simulink model "linemodel"  (R2016a)
settings: Solver=VariableStepAuto  StartTime=0.0  StopTime=inf  RelTol=1e-3
undefined symbols (not defined in the file): A, B, C, D
libraries: simulink x4
settings Model: Creator=Gray  LastModifiedBy=Gray

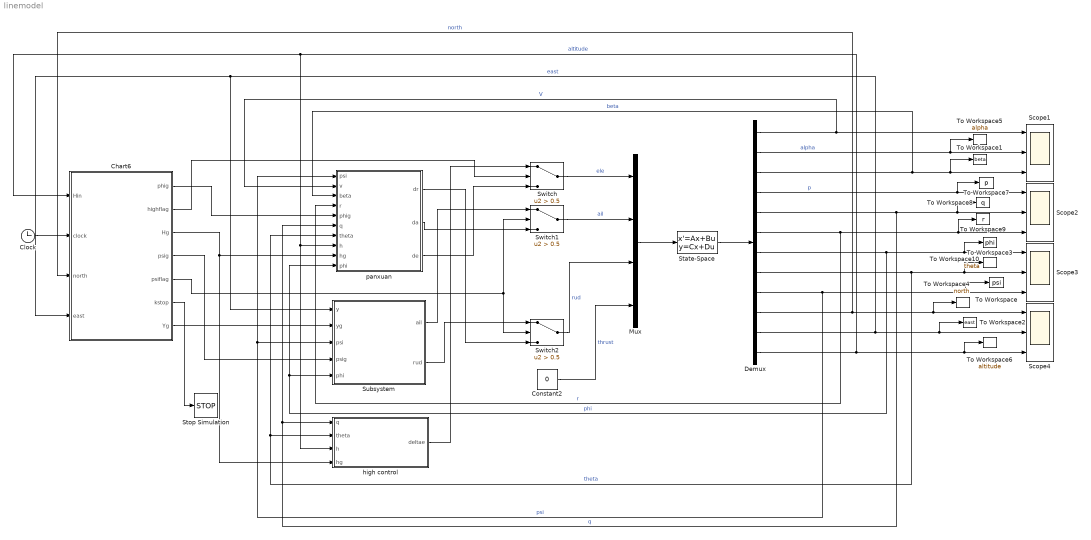
== system linemodel ==
  Chart6 : Stateflow chart  TreatAsAtomicUnit=on
  Clock : Clock
  Constant2 : Constant  Value=0
  Demux : Demux  Outputs=12
  Mux : Mux
  Scope{1..4} (4 alike) : Scope  NumInputPorts=3
  State-Space : StateSpace  A=A  B=B  C=C  D=D  X0=[20 0 0 0 0 0 0 0 0 0 0 0]
  Stop Simulation : Stop
  Subsystem : Subsystem
  Switch : Switch  Criteria=u2 > Threshold  Threshold=0.5
  Switch1 : Switch  Criteria=u2 > Threshold  Threshold=0.5
  Switch2 : Switch  Criteria=u2 > Threshold  Threshold=0.5
  To Workspace : ToWorkspace  VariableName=psi  SaveFormat=Timeseries  SampleTime=-1
  To Workspace1 : ToWorkspace  VariableName=beta  SaveFormat=Timeseries  SampleTime=-1
  To Workspace10 : ToWorkspace  VariableName=theta  SaveFormat=Timeseries  SampleTime=-1
  To Workspace2 : ToWorkspace  VariableName=east  SampleTime=-1
  To Workspace3 : ToWorkspace  VariableName=phi  SaveFormat=Timeseries  SampleTime=-1
  To Workspace4 : ToWorkspace  VariableName=north  SampleTime=-1
  To Workspace5 : ToWorkspace  VariableName=alpha  SaveFormat=Timeseries  SampleTime=-1
  To Workspace6 : ToWorkspace  VariableName=altitude  SaveFormat=Timeseries  SampleTime=-1
      settings: Save2DSignal=2-D array (concatenate along first dimension)
  To Workspace7 : ToWorkspace  VariableName=p  SaveFormat=Timeseries  SampleTime=-1
  To Workspace8 : ToWorkspace  VariableName=q  SaveFormat=Timeseries  SampleTime=-1
  To Workspace9 : ToWorkspace  VariableName=r  SaveFormat=Timeseries  SampleTime=-1
  high control : Subsystem
  panxuan : Subsystem
  wires:
  State-Space/1 -> Demux/1
  Mux/1 -> State-Space/1
  Demux/1 -> panxuan/2(v), Scope1/1  "V"
  Demux/2 -> To Workspace5/1, Scope1/2  "alpha"
  Demux/3 -> panxuan/3(beta), To Workspace1/1, Scope1/3  "beta"
  Demux/4 -> To Workspace7/1, Scope2/1  "p"
  Demux/5 -> panxuan/6(q), high control/1(q), To Workspace8/1, Scope2/2  "q"
  Demux/6 -> panxuan/4(r), To Workspace9/1, Scope2/3  "r"
  Demux/7 -> panxuan/10(phi), Subsystem/5(phi), To Workspace3/1, Scope3/1  "phi"
  Demux/8 -> high control/2(theta), panxuan/7(theta), To Workspace10/1, Scope3/2  "theta"
  Demux/9 -> Subsystem/3(psi), panxuan/1(psi), To Workspace/1, Scope3/3  "psi"
  Demux/10 -> Chart6/3(north), To Workspace4/1, Scope4/1  "north"
  Demux/11 -> Chart6/4(east), Subsystem/1(y), To Workspace2/1, Scope4/2  "east"
  Demux/12 -> Chart6/1(Hin), high control/3(h), panxuan/8(h), To Workspace6/1, Scope4/3  "altitude"
  Constant2/1 -> Mux/4  "thrust"
  Chart6/1(phig) -> panxuan/5(phig)
  Chart6/3(Hg) -> high control/4(hg), panxuan/9(hg)
  Chart6/7(Yg) -> Subsystem/2(yg)
  Chart6/4(psig) -> Subsystem/4(psig)
  Switch/1 -> Mux/1  "ele"
  Switch1/1 -> Mux/2  "ail"
  Switch2/1 -> Mux/3  "rud"
  high control/1(deltae) -> Switch/1
  panxuan/3(de) -> Switch/3
  Subsystem/1(ail) -> Switch1/1
  panxuan/2(da) -> Switch1/3
  Chart6/2(highflag) -> Switch/2
  Chart6/5(psiflag) -> Switch2/2, Switch1/2
  Clock/1 -> Chart6/2(clock)
  Chart6/6(kstop) -> Stop Simulation/1
  Subsystem/2(rud) -> Switch2/1
  panxuan/1(dr) -> Switch2/3

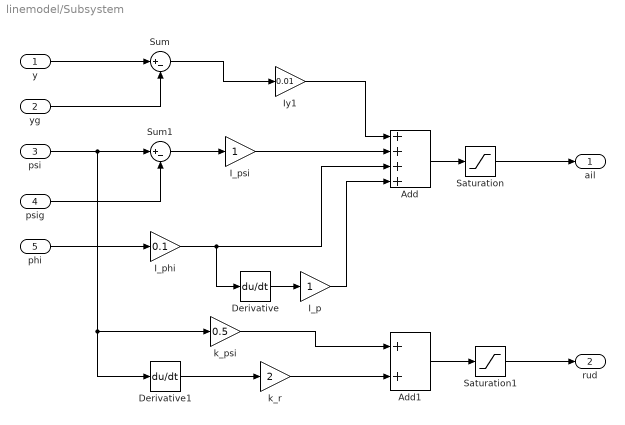
== system linemodel/Subsystem ==
  y : Inport
  yg : Inport  Port=2
  psi : Inport  Port=3
  psig : Inport  Port=4
  phi : Inport  Port=5
  Add : Sum  Inputs=++++
  Add1 : Sum
  Derivative : Derivative
  Derivative1 : Derivative
  I_p : Gain
  I_phi : Gain  Gain=0.1
  I_psi : Gain
  Iy1 : Gain  Gain=0.01
  Saturation : Saturate  UpperLimit=12  LowerLimit=-12
  Saturation1 : Saturate  UpperLimit=8  LowerLimit=-8
  Sum : Sum  Inputs=|+-
  Sum1 : Sum  Inputs=|+-
  k_psi : Gain  Gain=0.5
  k_r : Gain  Gain=2
  ail : Outport
  rud : Outport  Port=2
  wires:
  k_r/1 -> Add1/2
  k_psi/1 -> Add1/1
  Sum1/1 -> I_psi/1
  Add/1 -> Saturation/1
  Saturation/1 -> ail/1
  Add1/1 -> Saturation1/1
  Sum/1 -> Iy1/1
  Iy1/1 -> Add/1
  psi/1 -> Derivative1/1, k_psi/1, Sum1/1
  y/1 -> Sum/1
  psig/1 -> Sum1/2
  phi/1 -> I_phi/1
  I_phi/1 -> Derivative/1, Add/3
  Derivative/1 -> I_p/1
  Derivative1/1 -> k_r/1
  Saturation1/1 -> rud/1
  I_psi/1 -> Add/2
  I_p/1 -> Add/4
  yg/1 -> Sum/2

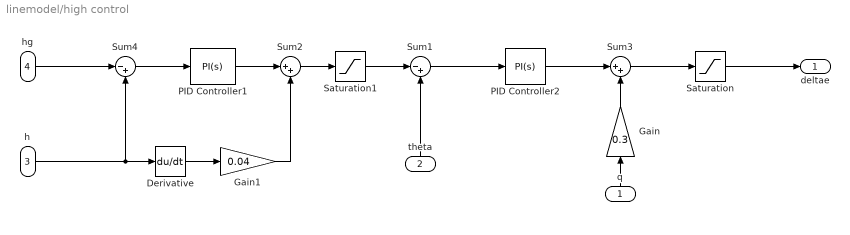
== system linemodel/high control ==
  q : Inport
  theta : Inport  Port=2
  h : Inport  Port=3
  hg : Inport  Port=4
  Derivative : Derivative
  Gain : Gain  Gain=0.3
  Gain1 : Gain  Gain=0.04
  PID Controller1 : simulink/Continuous/PID Controller  Controller=PI  TimeDomain=Continuous-time  SampleTime=-1  IntegratorMethod=Forward Euler  FilterMethod=Forward Euler  Form=Parallel  UseFilter=on  ControllerParametersSource=internal  P=0.03  I=0.0002  D=0  N=100  InitialConditionSource=internal  InitialConditionForIntegrator=0  InitialConditionForFilter=0  ExternalReset=none  LimitOutput=off  UpperSaturationLimit=inf  LowerSaturationLimit=-inf  LinearizeAsGain=on  AntiWindupMode=none  Kb=1  TrackingMode=off  Kt=1  PParamMin=[]  PParamMax=[]  IParamMin=[]  IParamMax=[]  DParamMin=[]  DParamMax=[]  NParamMin=[]  NParamMax=[]  KbParamMin=[]  KbParamMax=[]  KtParamMin=[]  KtParamMax=[]  POutMin=[]  POutMax=[]  IOutMin=[]  IOutMax=[]  DOutMin=[]  DOutMax=[]  NOutMin=[]  NOutMax=[]  KbOutMin=[]  KbOutMax=[]  KtOutMin=[]  KtOutMax=[]  IntegratorOutMin=[]  IntegratorOutMax=[]  FilterOutMin=[]  FilterOutMax=[]  SumOutMin=[]  SumOutMax=[]  SumI1OutMin=[]  SumI1OutMax=[]  SumI2OutMin=[]  SumI2OutMax=[]  SumI3OutMin=[]  SumI3OutMax=[]  SumDOutMin=[]  SumDOutMax=[]  SaturationOutMin=[]  SaturationOutMax=[]  IntegratorContinuousStateAttributes=''  IntegratorStateMustResolveToSignalObject=off  IntegratorRTWStateStorageClass=Auto  FilterContinuousStateAttributes=''  FilterStateMustResolveToSignalObject=off  FilterRTWStateStorageClass=Auto  DifferentiatorICPrevScaledInput=0  DifferentiatorOutMin=[]  DifferentiatorOutMax=[]
  PID Controller2 : simulink/Continuous/PID Controller  Controller=PI  TimeDomain=Continuous-time  SampleTime=-1  IntegratorMethod=Forward Euler  FilterMethod=Forward Euler  Form=Parallel  UseFilter=on  ControllerParametersSource=internal  P=0.5  I=0  D=0  N=100  InitialConditionSource=internal  InitialConditionForIntegrator=0  InitialConditionForFilter=0  ExternalReset=none  LimitOutput=off  UpperSaturationLimit=inf  LowerSaturationLimit=-inf  LinearizeAsGain=on  AntiWindupMode=none  Kb=1  TrackingMode=off  Kt=1  PParamMin=[]  PParamMax=[]  IParamMin=[]  IParamMax=[]  DParamMin=[]  DParamMax=[]  NParamMin=[]  NParamMax=[]  KbParamMin=[]  KbParamMax=[]  KtParamMin=[]  KtParamMax=[]  POutMin=[]  POutMax=[]  IOutMin=[]  IOutMax=[]  DOutMin=[]  DOutMax=[]  NOutMin=[]  NOutMax=[]  KbOutMin=[]  KbOutMax=[]  KtOutMin=[]  KtOutMax=[]  IntegratorOutMin=[]  IntegratorOutMax=[]  FilterOutMin=[]  FilterOutMax=[]  SumOutMin=[]  SumOutMax=[]  SumI1OutMin=[]  SumI1OutMax=[]  SumI2OutMin=[]  SumI2OutMax=[]  SumI3OutMin=[]  SumI3OutMax=[]  SumDOutMin=[]  SumDOutMax=[]  SaturationOutMin=[]  SaturationOutMax=[]  IntegratorContinuousStateAttributes=''  IntegratorStateMustResolveToSignalObject=off  IntegratorRTWStateStorageClass=Auto  FilterContinuousStateAttributes=''  FilterStateMustResolveToSignalObject=off  FilterRTWStateStorageClass=Auto  DifferentiatorICPrevScaledInput=0  DifferentiatorOutMin=[]  DifferentiatorOutMax=[]
  Saturation : Saturate  UpperLimit=9  LowerLimit=-9
  Saturation1 : Saturate  UpperLimit=15  LowerLimit=-15
  Sum1 : Sum  Inputs=|-+
  Sum2 : Sum  Inputs=|++
  Sum3 : Sum  Inputs=|++
  Sum4 : Sum  Inputs=|-+
  deltae : Outport
  wires:
  hg/1 -> Sum4/1
  Sum4/1 -> PID Controller1/1
  PID Controller1/1 -> Sum2/1
  Sum1/1 -> PID Controller2/1
  PID Controller2/1 -> Sum3/1
  Sum3/1 -> Saturation/1
  h/1 -> Derivative/1, Sum4/2
  theta/1 -> Sum1/2
  Gain/1 -> Sum3/2
  q/1 -> Gain/1
  Saturation/1 -> deltae/1
  Saturation1/1 -> Sum1/1
  Sum2/1 -> Saturation1/1
  Derivative/1 -> Gain1/1
  Gain1/1 -> Sum2/2

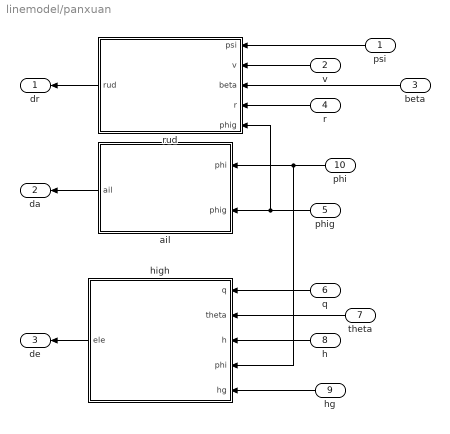
== system linemodel/panxuan ==
  psi : Inport
  v : Inport  Port=2
  beta : Inport  Port=3
  r : Inport  Port=4
  phig : Inport  Port=5
  q : Inport  Port=6
  theta : Inport  Port=7
  h : Inport  Port=8
  hg : Inport  Port=9
  phi : Inport  Port=10
  ail : Subsystem
  "high " : Subsystem
  rud : Subsystem
  dr : Outport
  da : Outport  Port=2
  de : Outport  Port=3
  wires:
  psi/1 -> rud/1(psi)
  "high "/1(ele) -> de/1
  beta/1 -> rud/3(beta)
  r/1 -> rud/4(r)
  ail/1(ail) -> da/1
  v/1 -> rud/2(v)
  phig/1 -> rud/5(phig), ail/2(phig)
  theta/1 -> "high "/2(theta)
  q/1 -> "high "/1(q)
  h/1 -> "high "/3(h)
  hg/1 -> "high "/5(hg)
  rud/1(rud) -> dr/1
  phi/1 -> "high "/4(phi), ail/1(phi)

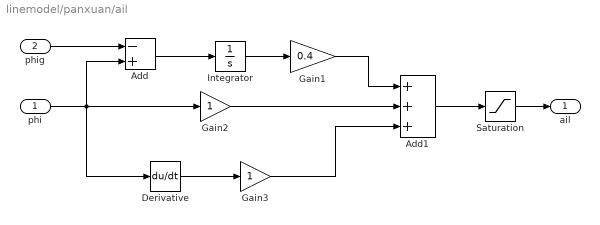
== system linemodel/panxuan/ail ==
  phi : Inport
  phig : Inport  Port=2
  Add : Sum  Inputs=-+
  Add1 : Sum  Inputs=+++
  Derivative : Derivative
  Gain1 : Gain  Gain=0.4
  Gain2 : Gain
  Gain3 : Gain
  Integrator : Integrator
  Saturation : Saturate  UpperLimit=12  LowerLimit=-12
  ail : Outport
  wires:
  phi/1 -> Derivative/1, Add/2, Gain2/1
  Add1/1 -> Saturation/1
  Add/1 -> Integrator/1
  Integrator/1 -> Gain1/1
  Saturation/1 -> ail/1
  phig/1 -> Add/1
  Derivative/1 -> Gain3/1
  Gain2/1 -> Add1/2
  Gain3/1 -> Add1/3
  Gain1/1 -> Add1/1

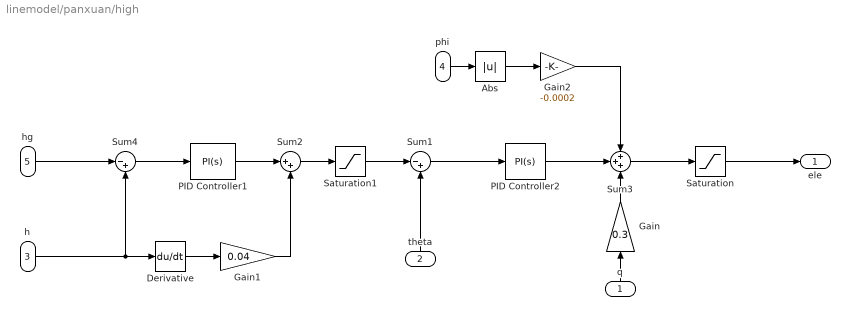
== system linemodel/panxuan/high  ==
  q : Inport
  theta : Inport  Port=2
  h : Inport  Port=3
  phi : Inport  Port=4
  hg : Inport  Port=5
  Abs : Abs
  Derivative : Derivative
  Gain : Gain  Gain=0.3
  Gain1 : Gain  Gain=0.04
  Gain2 : Gain  Gain=-0.0002
  PID Controller1 : simulink/Continuous/PID Controller  Controller=PI  TimeDomain=Continuous-time  SampleTime=-1  IntegratorMethod=Forward Euler  FilterMethod=Forward Euler  Form=Parallel  UseFilter=on  ControllerParametersSource=internal  P=0.03  I=0.0002  D=0  N=100  InitialConditionSource=internal  InitialConditionForIntegrator=0  InitialConditionForFilter=0  ExternalReset=none  LimitOutput=off  UpperSaturationLimit=inf  LowerSaturationLimit=-inf  LinearizeAsGain=on  AntiWindupMode=none  Kb=1  TrackingMode=off  Kt=1  PParamMin=[]  PParamMax=[]  IParamMin=[]  IParamMax=[]  DParamMin=[]  DParamMax=[]  NParamMin=[]  NParamMax=[]  KbParamMin=[]  KbParamMax=[]  KtParamMin=[]  KtParamMax=[]  POutMin=[]  POutMax=[]  IOutMin=[]  IOutMax=[]  DOutMin=[]  DOutMax=[]  NOutMin=[]  NOutMax=[]  KbOutMin=[]  KbOutMax=[]  KtOutMin=[]  KtOutMax=[]  IntegratorOutMin=[]  IntegratorOutMax=[]  FilterOutMin=[]  FilterOutMax=[]  SumOutMin=[]  SumOutMax=[]  SumI1OutMin=[]  SumI1OutMax=[]  SumI2OutMin=[]  SumI2OutMax=[]  SumI3OutMin=[]  SumI3OutMax=[]  SumDOutMin=[]  SumDOutMax=[]  SaturationOutMin=[]  SaturationOutMax=[]  IntegratorContinuousStateAttributes=''  IntegratorStateMustResolveToSignalObject=off  IntegratorRTWStateStorageClass=Auto  FilterContinuousStateAttributes=''  FilterStateMustResolveToSignalObject=off  FilterRTWStateStorageClass=Auto  DifferentiatorICPrevScaledInput=0  DifferentiatorOutMin=[]  DifferentiatorOutMax=[]
  PID Controller2 : simulink/Continuous/PID Controller  Controller=PI  TimeDomain=Continuous-time  SampleTime=-1  IntegratorMethod=Forward Euler  FilterMethod=Forward Euler  Form=Parallel  UseFilter=on  ControllerParametersSource=internal  P=0.5  I=0  D=0  N=100  InitialConditionSource=internal  InitialConditionForIntegrator=0  InitialConditionForFilter=0  ExternalReset=none  LimitOutput=off  UpperSaturationLimit=inf  LowerSaturationLimit=-inf  LinearizeAsGain=on  AntiWindupMode=none  Kb=1  TrackingMode=off  Kt=1  PParamMin=[]  PParamMax=[]  IParamMin=[]  IParamMax=[]  DParamMin=[]  DParamMax=[]  NParamMin=[]  NParamMax=[]  KbParamMin=[]  KbParamMax=[]  KtParamMin=[]  KtParamMax=[]  POutMin=[]  POutMax=[]  IOutMin=[]  IOutMax=[]  DOutMin=[]  DOutMax=[]  NOutMin=[]  NOutMax=[]  KbOutMin=[]  KbOutMax=[]  KtOutMin=[]  KtOutMax=[]  IntegratorOutMin=[]  IntegratorOutMax=[]  FilterOutMin=[]  FilterOutMax=[]  SumOutMin=[]  SumOutMax=[]  SumI1OutMin=[]  SumI1OutMax=[]  SumI2OutMin=[]  SumI2OutMax=[]  SumI3OutMin=[]  SumI3OutMax=[]  SumDOutMin=[]  SumDOutMax=[]  SaturationOutMin=[]  SaturationOutMax=[]  IntegratorContinuousStateAttributes=''  IntegratorStateMustResolveToSignalObject=off  IntegratorRTWStateStorageClass=Auto  FilterContinuousStateAttributes=''  FilterStateMustResolveToSignalObject=off  FilterRTWStateStorageClass=Auto  DifferentiatorICPrevScaledInput=0  DifferentiatorOutMin=[]  DifferentiatorOutMax=[]
  Saturation : Saturate  UpperLimit=9  LowerLimit=-9
  Saturation1 : Saturate  UpperLimit=15  LowerLimit=-15
  Sum1 : Sum  Inputs=|-+
  Sum2 : Sum  Inputs=|++
  Sum3 : Sum  Inputs=+++
  Sum4 : Sum  Inputs=|-+
  ele : Outport
  wires:
  hg/1 -> Sum4/1
  Sum4/1 -> PID Controller1/1
  PID Controller1/1 -> Sum2/1
  Sum1/1 -> PID Controller2/1
  Sum3/1 -> Saturation/1
  h/1 -> Derivative/1, Sum4/2
  theta/1 -> Sum1/2
  q/1 -> Gain/1
  Saturation/1 -> ele/1
  Saturation1/1 -> Sum1/1
  Sum2/1 -> Saturation1/1
  Derivative/1 -> Gain1/1
  Gain1/1 -> Sum2/2
  PID Controller2/1 -> Sum3/2
  Gain/1 -> Sum3/3
  phi/1 -> Abs/1
  Abs/1 -> Gain2/1
  Gain2/1 -> Sum3/1

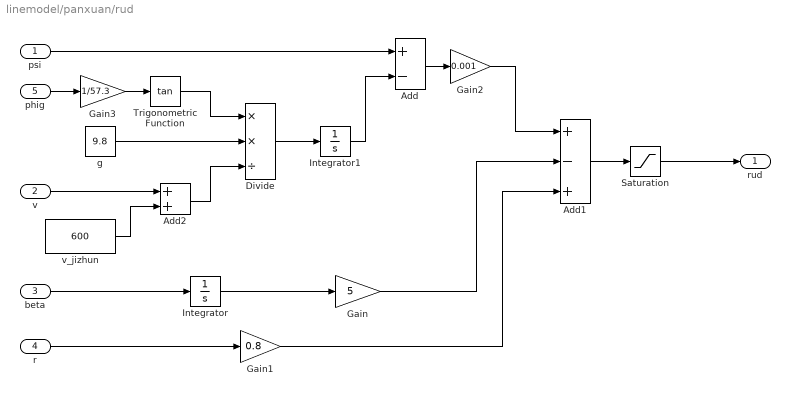
== system linemodel/panxuan/rud ==
  psi : Inport
  v : Inport  Port=2
  beta : Inport  Port=3
  r : Inport  Port=4
  phig : Inport  Port=5
  Add : Sum  Inputs=+-
  Add1 : Sum  Inputs=+-+
  Add2 : Sum
  Divide : Product  Inputs=**/
  Gain : Gain  Gain=5
  Gain1 : Gain  Gain=0.8
  Gain2 : Gain  Gain=0.001
  Gain3 : Gain  Gain=1/57.3
  Integrator : Integrator
  Integrator1 : Integrator
  Saturation : Saturate  UpperLimit=8  LowerLimit=-8
  Trigonometric Function : Trigonometry  Operator=tan
  g : Constant  Value=9.8
  v_jizhun : Constant  Value=600
  rud : Outport
  wires:
  Saturation/1 -> rud/1
  Add1/1 -> Saturation/1
  Trigonometric Function/1 -> Divide/1
  g/1 -> Divide/2
  psi/1 -> Add/1
  Add/1 -> Gain2/1
  r/1 -> Gain1/1
  Divide/1 -> Integrator1/1
  Integrator1/1 -> Add/2
  Add2/1 -> Divide/3
  v/1 -> Add2/1
  v_jizhun/1 -> Add2/2
  Gain1/1 -> Add1/3
  Integrator/1 -> Gain/1
  beta/1 -> Integrator/1
  Gain2/1 -> Add1/1
  Gain/1 -> Add1/2
  phig/1 -> Gain3/1
  Gain3/1 -> Trigonometric Function/1

== stateflow chart linemodel/Chart6 ==
  state panxuan
    entry:highflag=0;
    Hg=200;psig=0;psiflag=0;
    Yg=100;phig=10;
    exit:tt3=clock;
  state pingfei1
    entry:highflag=1;
    Hg=-200;psig=0;psiflag=1;
    Yg=0;phig=0;
  state xiahua
    entry:highflag=1;
    Hg=200;psig=0;psiflag=1;
    Yg=0;phig=0;
    exit: tt2=clock;
  state pingfei
    entry:highflag=1;
    Hg=0;psig=0;psiflag=1;
    Yg=0;phig=0;
  state pasheng
    entry:highflag=1;
    Hg=-200;psig=0;psiflag=1;
    Yg=0;phig=0;
    exit: tt1=clock;
  state pingfei4
    entry:highflag=1;
    Hg=200;psig=0;psiflag=1;
    Yg=100;phig=0;
  state stop
    entry:kstop=1;
  state pingfei3
    entry:highflag=1;
    Hg=200;psig=0;psiflag=1;
    Yg=0;phig=0;
  state cepian
    entry:highflag=1;
    Hg=200;psig=0;psiflag=1;
    Yg=100;phig=0;
  (default) -> pingfei
  pingfei1 -> xiahua : [clock>tt1+40]
  panxuan -> stop : [clock>tt3+1000]
  pingfei4 -> panxuan : [sqrt((north-5000)^2+(east-Yg)^2)<100]
  pasheng -> pingfei1 : [(Hin<=-195)&&(Hin>=-205)]
  xiahua -> pingfei3 : [(Hin>=195)&&(Hin<=205)]
  pingfei -> pasheng : [clock>20]
  cepian -> pingfei4 : [(east>95)&&(east<105)]
  pingfei3 -> cepian : [clock>tt2+20]
  data: Hin input double; phig output double; highflag output double; clock input double; Hg output double; psig output double; psiflag output double; kstop output double; north input double; east input double; Yg output double; tt1 local double; tt2 local double; tt3 local double
